simulink model "model1"  (R2023a)
settings: Solver=VariableStepAuto  StartTime=0.0  StopTime=10.0  RelTol=1e-3
values from neighbouring files (symbols this model uses):
  A = [0, 1, 0, 0 ... (first row only)    [e01.m]
  B = [0, 0 ... (first row only)    [e01.m]
  C = [1, 0, 0, 0 ... (first row only)    [e01.m]
  D = [0, 0 ... (first row only)    [e01.m]
settings Model: Creator=Anirvan Krishna  LastModifiedBy=Anirvan Krishna

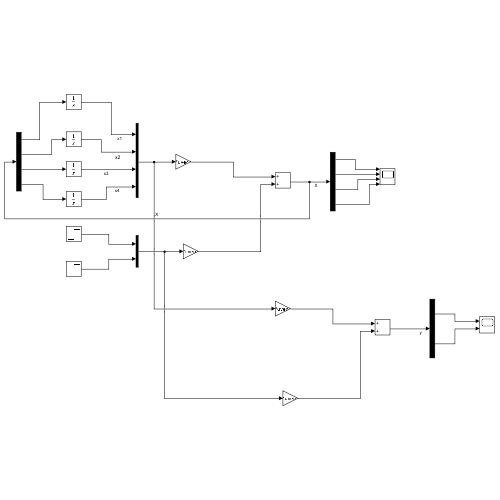
[thumbnail: Simulink's stored preview of the top-level diagram]
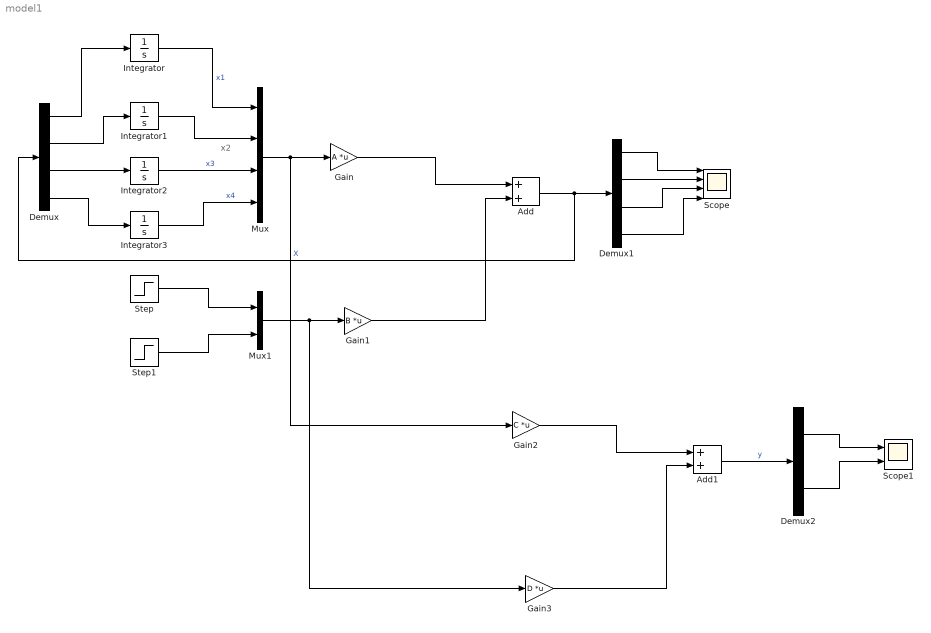
== system model1 ==
  note: x2
  Add : Sum
  Add1 : Sum
  Demux : Demux
  Demux1 : Demux
  Demux2 : Demux  Outputs=2
  Gain : Gain  Gain=A  Multiplication=Matrix(K*u) (u vector)
  Gain1 : Gain  Gain=B  Multiplication=Matrix(K*u) (u vector)
  Gain2 : Gain  Gain=C  Multiplication=Matrix(K*u) (u vector)
  Gain3 : Gain  Gain=D  Multiplication=Matrix(K*u) (u vector)
  Integrator{,1..3} (4 alike) : Integrator
  Mux : Mux
  Mux1 : Mux  Inputs=2
  Scope : Scope  NumInputPorts=4
  Scope1 : Scope  NumInputPorts=2
  Step : Step  Time=0  SampleTime=0
  Step1 : Step  Time=0  SampleTime=0
  wires:
  Demux/1 -> Integrator/1
  Demux/2 -> Integrator1/1
  Demux/3 -> Integrator2/1
  Demux/4 -> Integrator3/1
  Integrator/1 -> Mux/1  "x1"
  Integrator1/1 -> Mux/2
  Integrator2/1 -> Mux/3  "x3"
  Integrator3/1 -> Mux/4  "x4"
  Gain1/1 -> Add/2
  Add/1 -> Demux1/1, Demux/1  "X"
  Step/1 -> Mux1/1
  Step1/1 -> Mux1/2
  Demux1/1 -> Scope/1
  Demux1/2 -> Scope/2
  Demux1/3 -> Scope/3
  Demux1/4 -> Scope/4
  Gain/1 -> Add/1
  Mux/1 -> Gain2/1, Gain/1
  Demux2/2 -> Scope1/2
  Gain3/1 -> Add1/2
  Gain2/1 -> Add1/1
  Mux1/1 -> Gain3/1, Gain1/1
  Add1/1 -> Demux2/1  "y"
  Demux2/1 -> Scope1/1
